simulink subsystem "BEVController_Inputs_Random_refsub"  (R2025a)
settings: Solver=VariableStepAuto  StartTime=0.0  StopTime=10.0  RelTol=1e-3
libraries: simulink x1
settings Model: Creator=isaacito  LastModifiedBy=isaacito

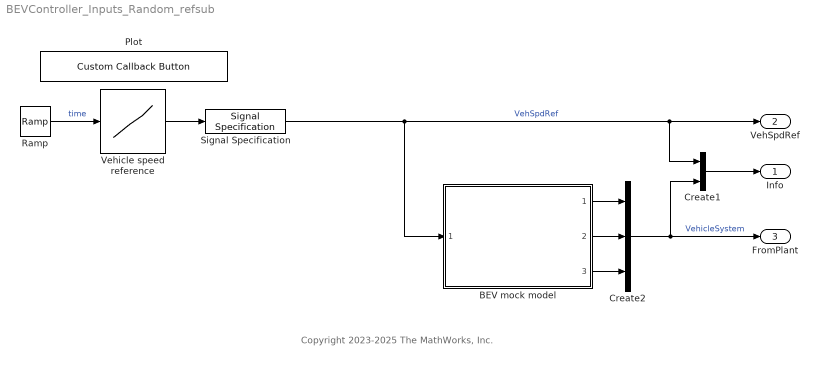
== system BEVController_Inputs_Random_refsub ==
  note: Copyright 2023-2025 The MathWorks, Inc.
  BEV mock model : Subsystem  ReferencedSubsystem=BEV_MockModel_refsub
  Create1 : BusCreator  Inputs=2
  Create2 : BusCreator  Inputs=3
  Plot : CustomCallbackButton  Configuration="{\"components\":[{\"name\":\"BackgroundImageComponent\",\"settings\":{\"image\":{\"size\":[0,0],\"src\":\"default\",\"srcOrientation\":\"Right\"},\"position\":[0,0,1,1]}},{\"name\":\"ButtonStateComponent\",\"settings\":{\"buttonType\":\"momentary\",\"clickFcn\":\"SignalTool2.plotSimulink1DLookupTableBlock(gcs + \\\"\\/Vehicle speed reference\\\", DivsionType=\\\"InterpolationInterval\\\", InterpolationInterval=0.2)\",\"onValue\":1,\"position\":[0,0,1,1],\"pressDelay\":\"500\",\"pressFcn\":\"\",\"repeatInterval\":\"0\",\"states\":[{\"horizontalAlignment\":\"center\",\"image\":{\"position\":[0,0,1,1],\"size\":[1,1],\"src\":\"default\",\"srcOrientation\":\"Right\"},\"label\":{\"color\":[0.01176470588,0.01176470588,0.01176470588,1],\"icon\":{\"size\":[0,0],\"src\":\"default\",\"srcOrientation\":\"Right\"},\"iconOffset\":0,\"iconPlacement\":\"left\",\"opacity\":1,\"show\":true,\"text\":{\"content\":\"Vehicle speed reference\",\"font\":\"Helvetica\"}},\"labelOffset\":[0,0],\"verticalAlignment\":\"middle\"},{\"horizontalAlignment\":\"center\",\"image\":{\"position\":[0,0,1,1],\"size\":[1,1],\"src\":\"default\",\"srcOrientation\":\"Right\"},\"label\":{\"color\":[0.01176470588,0.01176470588,0.01176470588,1],\"icon\":{\"size\":[0,0],\"src\":\"default\",\"srcOrientation\":\"Right\"},\"iconOffset\":0,\"iconPlacement\":\"left\",\"opacity\":1,\"show\":true,\"text\":{\"content\":\"Vehicle speed reference\",\"font\":\"Helvetica\"}},\"labelOffset\":[0,0],\"verticalAlignment\":\"middle\"},{\"horizontalAlignment\":\"center\",\"image\":{\"position\":[0,0,1,1],\"size\":[1,1],\"src\":\"default\",\"srcOrientation\":\"Right\"},\"label\":{\"color\":[0.01176470588,0.01176470588,0.01176470588,1],\"icon\":{\"size\":[0,0],\"src\":\"default\",\"srcOrientation\":\"Right\"},\"iconOffset\":0,\"iconPlacement\":\"left\",\"opacity\":1,\"show\":true,\"text\":{\"content\":\"Vehicle speed reference\",\"font\":\"Helvetica\"}},\"labelOffset\":[0,0],\"verticalAlignment\":\"middle\"},{\"horizontalAlignment\":\"center\",\"image\":{\"position\":[0,0,1,1],\"size\":[1,1],\"src\":\"default\",\"srcOrientation\":\"Right\"},\"label\":{\"color\":[0.01176470588,0.01176470588,0.01176470588,1],\"icon\":{\"size\":[0,0],\"src\":\"default\",\"srcOrientation\":\"Right\"},\"iconOffset\":0,\"iconPlacement\":\"left\",\"opacity\":1,\"show\":true,\"text\":{\"content\":\"Vehicle speed reference\",\"font\":\"Helvetica\"}},\"labelOffset\":[0,0],\"verticalAlignment\":\"middle\"}]}},{\"name\":\"ForegroundImageComponent\",\"settings\":{\"image\":{\"size\":[0,0],\"src\":\"default\",\"srcOrientation\":\"Right\"},\"isForeground\":1,\"position\":[0,0,1,1]}}],\"derived\":{\"blockParameters\":{\"AutoActivate\":true,\"ButtonText\":\"Vehicle speed reference\",\"ButtonType\":\"Momentary\",\"ClickFcn\":\"SignalTool2.plotSimulink1DLookupTableBlock(gcs + \\\"\\/Vehicle speed reference\\\", DivsionType=\\\"InterpolationInterval\\\", InterpolationInterval=0.2)\",\"OnValue\":1,\"PressDelay\":\"500\",\"PressFcn\":\"\",\"RepeatInterval\":\"0\",\"fixedAspectRatio\":\"off\"}},\"settings\":{\"BindingType\":\"standalone\",\"autoActivate\":true,\"backgroundColor\":[244,244,244,1],\"backgroundOffset\":0.2,\"backgroundOpacity\":1,\"fixedAspectRatio\":\"off\",\"foregroundColor\":[0.01176470588,0.01176470588,0.01176470588,1],\"migratedFromLegacy\":true,\"useBackgroundColor\":true,\"variant\":\"callback\",\"version\":\"R2025a\"},\"type\":\"Button\"}"  CustomBackgroundColor="{\"color\":[0.9568627451,0.9568627451,0.9568627451],\"show\":true}"
  Ramp : simulink/Sources/Ramp  slope=1  start=0  InitialOutput=0
      settings: AttributesFormatString=|
      | Slope: %<slope>
      | Start time: %<start>
      | Initial output: %<InitialOutput>
  Signal Specification : SignalSpecification  Unit=km/h
  Vehicle speed reference : Lookup_n-D  NumberOfTableDimensions=1  BreakpointsForDimension1=[0; 50; 100; 120; 141; 162; 168; 238; 308; 311; 401; 491; 493; 521.5; 550; 555; 635.5; 716; 718; 770; 822; 829; 935.5; 1042; 1047; 1105; 1163; 1169; 1295.5; 1422; 1426; 1501; 1576; 1581; 1661; 1741; 1761; 1766; 1771]  Table=[0; 0; 0; 63; 63; 63; 100; 100; 100; 71; 71; 71; 74; 74; 74; 42; 42; 42; 83; 83; 83; 65; 65; 65; 66; 66; 66; 57; 57; 57; 94; 94; 94; 80; 80; 80; 0; 0; 0]  InterpMethod=Akima spline  InternalRulePriority=Speed  RndMeth=Simplest
  Info : Outport
  VehSpdRef : Outport  Port=2
  FromPlant : Outport  Port=3
  wires:
  Create2/1 -> FromPlant/1, Create1/2  "VehicleSystem"
  Create1/1 -> Info/1
  BEV mock model/1 -> Create2/1
  BEV mock model/2 -> Create2/2
  BEV mock model/3 -> Create2/3
  Ramp/1 -> Vehicle speed reference/1  "time"
  Vehicle speed reference/1 -> Signal Specification/1
  Signal Specification/1 -> BEV mock model/1, Create1/1, VehSpdRef/1  "VehSpdRef"
